simulink model "CVAmdl"  (R2021a)
settings: Solver=ode45  StartTime=0.0  StopTime=15  RelTol=1e-3
values from neighbouring files (symbols this model uses):
  alpha = 1    [CVAmdl_params.m]
  beta = 1    [CVAmdl_params.m]
  gamma = 0.7    [CVAmdl_params.m]
  HR_eq = 70    [CVAmdl_params.m]
  m = -0.09    [CVAmdl_params.m]
  MAP_eq = 90    [CVAmdl_params.m]
  R0 = 350    [CVAmdl_params.m]
  RAP = 5    [CVAmdl_params.m]
  S_p = 0.01    [CVAmdl_params.m]
  S_r = 0.01    [CVAmdl_params.m]
  SV = 0.097    [CVAmdl_params.m]
  T = 10    [CVAmdl_params.m]
  t1 = 0.01    [CVAmdl_params.m]
  t2 = 0.01    [CVAmdl_params.m]
  TPR_eq = 12.5    [CVAmdl_params.m]
settings Model: Creator=nakyani  LastModifiedBy=Kyrie

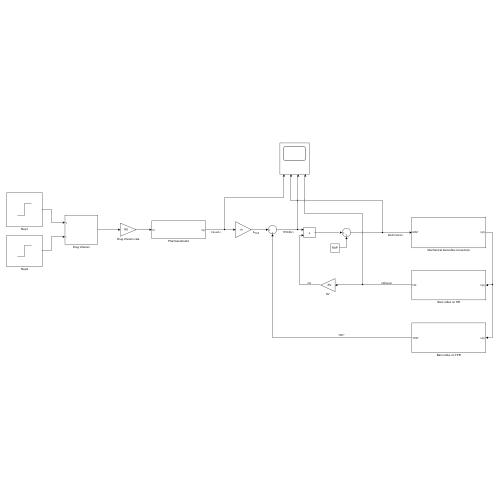
[thumbnail: Simulink's stored preview of the top-level diagram]
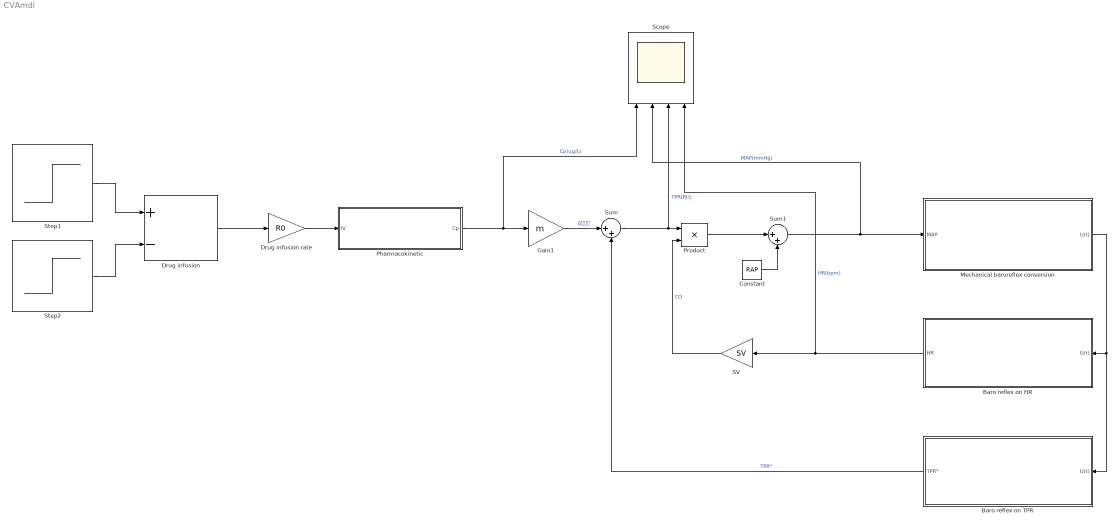
== system CVAmdl ==
  Baro reflex on HR : Subsystem
  Baro reflex on TPR : Subsystem
  Constant : Constant  Value=RAP
  Drug infusion : Sum  Inputs=+-
  Drug infusion rate : Gain  Gain=R0
  Gain1 : Gain  Gain=m
  Mechanical baroreflex conversion : Subsystem
  Pharmacokinetic : Subsystem
  Product : Product
  SV : Gain  Gain=SV
  Scope : Scope  NumInputPorts=4
  Step1 : Step  Time=0  SampleTime=0
  Step2 : Step  Time=T  SampleTime=0
  Sum : Sum  Inputs=|++
  Sum1 : Sum  Inputs=|++
  wires:
  Step1/1 -> Drug infusion/1
  Step2/1 -> Drug infusion/2
  Drug infusion/1 -> Drug infusion rate/1
  Drug infusion rate/1 -> Pharmacokinetic/1(IV)
  Pharmacokinetic/1(Cp) -> Scope/1, Gain1/1  "Cp(ug/L)"
  Baro reflex on TPR/1(TPR*) -> Sum/2  "TPR*"
  Baro reflex on HR/1(HR) -> Scope/4, SV/1  "HR(bpm)"
  Sum/1 -> Product/1, Scope/3  "TPR(RU)"
  SV/1 -> Product/2  "CO"
  Product/1 -> Sum1/1
  Sum1/1 -> Mechanical baroreflex conversion/1(MAP), Scope/2  "MAP(mmHg)"
  Mechanical baroreflex conversion/1(U(t)) -> Baro reflex on TPR/1(U(t)), Baro reflex on HR/1(U(t))
  Constant/1 -> Sum1/2
  Gain1/1 -> Sum/1  "Δ𝑇𝑃𝑅"

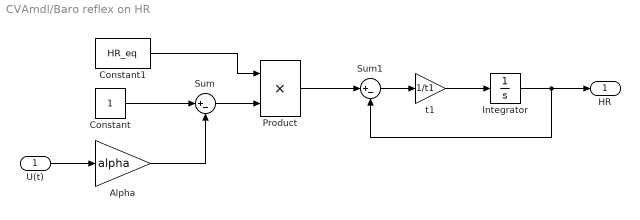
== system CVAmdl/Baro reflex on HR ==
  U(t) : Inport
  Alpha : Gain  Gain=alpha
  Constant : Constant
  Constant1 : Constant  Value=HR_eq
  Integrator : Integrator  InitialCondition=HR_eq
  Product : Product
  Sum : Sum  Inputs=|+-
  Sum1 : Sum  Inputs=|+-
  t1 : Gain  Gain=1/t1
  HR : Outport
  wires:
  U(t)/1 -> Alpha/1
  Alpha/1 -> Sum/2
  Constant/1 -> Sum/1
  Constant1/1 -> Product/1
  Sum/1 -> Product/2
  Product/1 -> Sum1/1
  Sum1/1 -> t1/1
  t1/1 -> Integrator/1
  Integrator/1 -> Sum1/2, HR/1

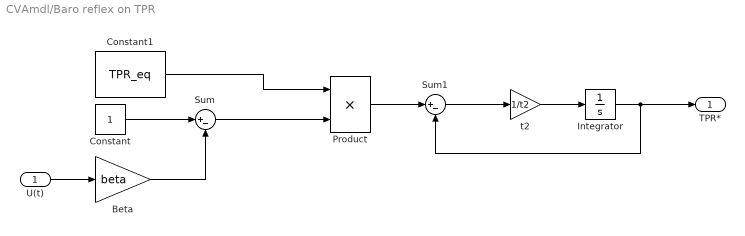
== system CVAmdl/Baro reflex on TPR ==
  U(t) : Inport
  Beta : Gain  Gain=beta
  Constant : Constant
  Constant1 : Constant  Value=TPR_eq
  Integrator : Integrator  InitialCondition=TPR_eq
  Product : Product
  Sum : Sum  Inputs=|+-
  Sum1 : Sum  Inputs=|+-
  t2 : Gain  Gain=1/t2
  TPR* : Outport
  wires:
  U(t)/1 -> Beta/1
  Beta/1 -> Sum/2
  Constant/1 -> Sum/1
  Sum/1 -> Product/2
  Product/1 -> Sum1/1
  Sum1/1 -> t2/1
  t2/1 -> Integrator/1
  Integrator/1 -> Sum1/2, TPR*/1
  Constant1/1 -> Product/1

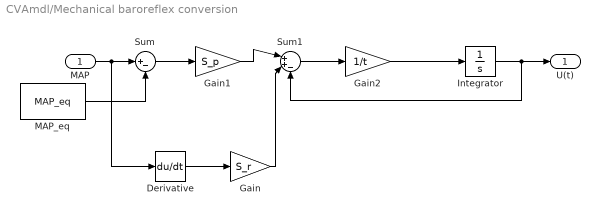
== system CVAmdl/Mechanical baroreflex conversion ==
  MAP : Inport
  Derivative : Derivative
  Gain : Gain  Gain=S_r
  Gain1 : Gain  Gain=S_p
  Gain2 : Gain  Gain=1/t
  Integrator : Integrator
  MAP_eq : Constant  Value=MAP_eq
  Sum : Sum  Inputs=|+-
  Sum1 : Sum  Inputs=|++-
  U(t) : Outport
  wires:
  MAP/1 -> Derivative/1, Sum/1
  Sum/1 -> Gain1/1
  Gain1/1 -> Sum1/1
  Sum1/1 -> Gain2/1
  MAP_eq/1 -> Sum/2
  Derivative/1 -> Gain/1
  Gain/1 -> Sum1/2
  Gain2/1 -> Integrator/1
  Integrator/1 -> Sum1/3, U(t)/1

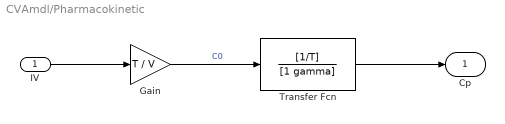
== system CVAmdl/Pharmacokinetic ==
  IV : Inport
  Gain : Gain  Gain=T / V
  Transfer Fcn : TransferFcn  Numerator=[1/T]  Denominator=[1 gamma]
  Cp : Outport
  wires:
  IV/1 -> Gain/1
  Gain/1 -> Transfer Fcn/1  "C0"
  Transfer Fcn/1 -> Cp/1
